simulink library "partitionedLifitngBdy_cl"  (R2018b)
settings: Solver=VariableStepAuto  StartTime=0.0  StopTime=10.0  RelTol=1e-3
values from neighbouring files (symbols this model uses):
  fluidDensity = 1    [partitionedLifitngBdy_ts.m]
undefined symbols (not defined in the file or in its folder): aeroStruct
libraries: vrlib x2, vectorNormalizer_ul x2, eulAng2RotMat_ul x1, alphaBeta_ul x1, surfaceCoefficients_ul x1
settings Model: Creator=mcobb  LastModifiedBy=asiddiq2

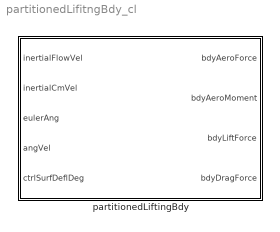
== system partitionedLifitngBdy_cl ==
  partitionedLiftingBdy : Subsystem  mask{rho_fluid=fluidDensity, aero_struct=aeroStruct}
      mask prompts: rho_fluid "Fluid density"; aero_struct "Structure containing AVL data"
      mask DialogControl ParameterGroupVar Prompt: Environment
      mask DialogControl Container3 Prompt: Fluid dynamic properties

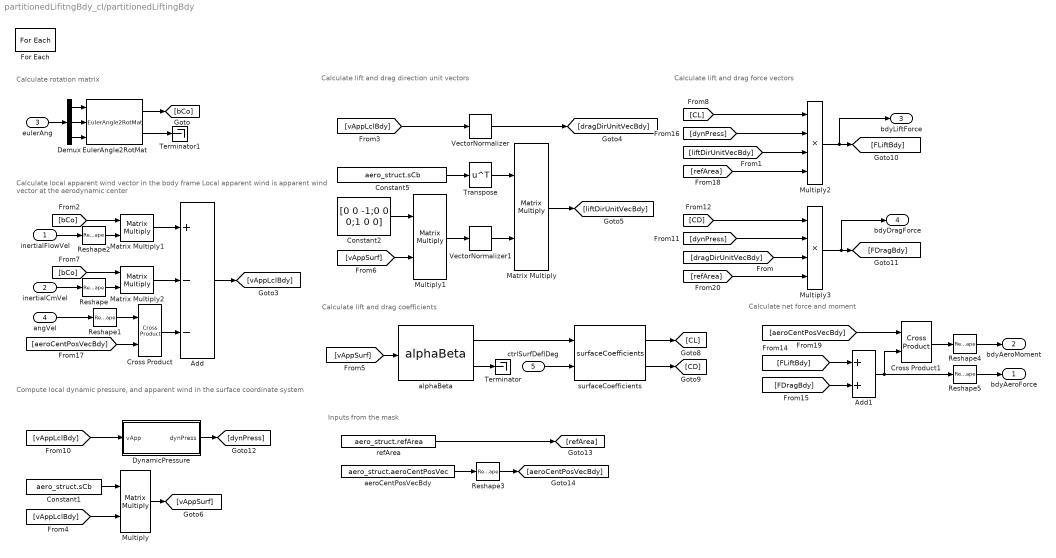
== system partitionedLifitngBdy_cl/partitionedLiftingBdy ==
  note: Calculate rotation matrix
  note: Calculate net force and moment
  note: Calculate lift and drag force vectors
  note: Calculate lift and drag coefficients
  note: Compute local dynamic pressure,
      | and apparent wind in the surface coordinate system
  note: Inputs from the mask
  note: Calculate lift and drag direction unit vectors
  note: Calculate local apparent wind vector in the body frame
      | Local apparent wind is apparent wind vector at the aerodynamic center
  inertialFlowVel : Inport
  inertialCmVel : Inport  Port=2
  eulerAng : Inport  Port=3
  angVel : Inport  Port=4
  ctrlSurfDeflDeg : Inport  Port=5  Partition=on  PartitionDimension=1  PartitionWidth=1  PartitionOffset=0
  Add : Sum  Inputs=+--
  Add1 : Sum
  Constant1 : Constant  Value=aero_struct.sCb  VectorParams1D=off
  Constant2 : Constant  Value=[0 0 -1;0 0 0;1 0 0]
  Constant5 : Constant  Value=aero_struct.sCb  VectorParams1D=off
  Cross Product : vrlib/Utilities/Cross Product
      settings: SourceProductBaseCode=VR
  Cross Product1 : vrlib/Utilities/Cross Product
      settings: SourceProductBaseCode=VR
  Demux : Demux  Outputs=3
  DynamicPressure : Subsystem  mask{rho=rho_fluid}
      mask prompts: rho "Fluid density"
  EulerAngle2RotMat : eulAng2RotMat_ul/EulerAngle2RotMat  SystemSampleTime=-1
  For Each : ForEach  DisableCoverage=on  IterateSubsysMaskParameter=off,on  SubsysMaskParameterIterationDimension=1,2  IndexMode=One-based
  Matrix Multiply : Product  Multiplication=Matrix(*)
  Matrix Multiply1 : Product  Multiplication=Matrix(*)
  Matrix Multiply2 : Product  Multiplication=Matrix(*)
  Multiply : Product  Multiplication=Matrix(*)
  Multiply1 : Product  Multiplication=Matrix(*)
  Multiply2 : Product  Inputs=4
  Multiply3 : Product  Inputs=4
  Reshape{,1..5} (6 alike) : Reshape  OutputDimensionality=Column vector (2-D)
  Terminator : Terminator
  Terminator1 : Terminator
  Transpose : Math  Operator=transpose  SaturateOnIntegerOverflow=on
  "VectorNormalizer " : vectorNormalizer_ul/VectorNormalizer   SystemSampleTime=-1
  VectorNormalizer1 : vectorNormalizer_ul/VectorNormalizer   SystemSampleTime=-1
  aeroCentPosVecBdy : Constant  Value=aero_struct.aeroCentPosVec  VectorParams1D=off
  alphaBeta : alphaBeta_ul/alphaBeta  SystemSampleTime=-1
  refArea : Constant  Value=aero_struct.refArea  VectorParams1D=off
  surfaceCoefficients : surfaceCoefficients_ul/surfaceCoefficients  CLval=aero_struct.CL  CDval=aero_struct.CD  alp=aero_struct.alpha  GainCL=aero_struct.GainCL  GainCD=aero_struct.GainCD  maxCsDefUp=aero_struct.MaxCtrlDeflUp  maxCsDefDn=aero_struct.MaxCtrlDeflDn
  bdyAeroForce : Outport  ConcatenationDimension=2
  bdyAeroMoment : Outport  Port=2  PortDimensions=[3 1]  ConcatenationDimension=2
  bdyLiftForce : Outport  Port=3  ConcatenationDimension=2
  bdyDragForce : Outport  Port=4  ConcatenationDimension=2
  wires:
  Cross Product/1 -> Add/3
  inertialFlowVel/1 -> Reshape2/1
  inertialCmVel/1 -> Reshape/1
  angVel/1 -> Reshape1/1
  Reshape1/1 -> Cross Product/1
  [aeroCentPosVecBdy] -> Cross Product/2
  Add/1 -> [vAppLclBdy]
  [vAppLclBdy] -> "VectorNormalizer "/1
  "VectorNormalizer "/1 -> [dragDirUnitVecBdy]
  Constant1/1 -> Multiply/1
  [vAppLclBdy] -> Multiply/2
  Multiply/1 -> [vAppSurf]
  [vAppSurf] -> alphaBeta/1
  [vAppSurf] -> Multiply1/2
  Constant2/1 -> Multiply1/1
  Multiply1/1 -> VectorNormalizer1/1
  alphaBeta/2 -> Terminator/1
  surfaceCoefficients/1 -> [CL]
  surfaceCoefficients/2 -> [CD]
  [CL] -> Multiply2/1
  DynamicPressure/1(dynPress) -> [dynPress]
  [liftDirUnitVecBdy] -> Multiply2/3
  [vAppLclBdy] -> DynamicPressure/1(vApp)
  Multiply2/1 -> bdyLiftForce/1, [FLiftBdy]
  Multiply3/1 -> bdyDragForce/1, [FDragBdy]
  [dragDirUnitVecBdy] -> Multiply3/3
  [dynPress] -> Multiply3/2
  [CD] -> Multiply3/1
  Add1/1 -> Reshape5/1, Cross Product1/2
  [FDragBdy] -> Add1/2
  [FLiftBdy] -> Add1/1
  Constant5/1 -> Transpose/1
  Matrix Multiply/1 -> [liftDirUnitVecBdy]
  Transpose/1 -> Matrix Multiply/1
  VectorNormalizer1/1 -> Matrix Multiply/2
  [dynPress] -> Multiply2/2
  Cross Product1/1 -> Reshape4/1
  aeroCentPosVecBdy/1 -> Reshape3/1
  [refArea] -> Multiply2/4
  [refArea] -> Multiply3/4
  [aeroCentPosVecBdy] -> Cross Product1/1
  refArea/1 -> [refArea]
  Reshape3/1 -> [aeroCentPosVecBdy]
  Reshape4/1 -> bdyAeroMoment/1
  Reshape5/1 -> bdyAeroForce/1
  ctrlSurfDeflDeg/1 -> surfaceCoefficients/2
  alphaBeta/1 -> surfaceCoefficients/1
  eulerAng/1 -> Demux/1
  Demux/1 -> EulerAngle2RotMat/1
  Demux/2 -> EulerAngle2RotMat/2
  Demux/3 -> EulerAngle2RotMat/3
  EulerAngle2RotMat/1 -> [bCo]
  EulerAngle2RotMat/2 -> Terminator1/1
  Reshape2/1 -> Matrix Multiply1/2
  Matrix Multiply1/1 -> Add/1
  [bCo] -> Matrix Multiply1/1
  Reshape/1 -> Matrix Multiply2/2
  Matrix Multiply2/1 -> Add/2
  [bCo] -> Matrix Multiply2/1

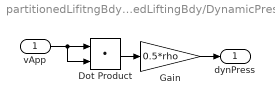
== system partitionedLifitngBdy_cl/partitionedLiftingBdy/DynamicPressure ==
  vApp : Inport
  Dot Product : DotProduct  InputSameDT=on  OutDataTypeStr=Inherit: Inherit via internal rule
  Gain : Gain  Gain=0.5*rho
  dynPress : Outport
  wires:
  Dot Product/1 -> Gain/1
  vApp/1 -> Dot Product/1, Dot Product/2
  Gain/1 -> dynPress/1
